simulink model "obs_student"  (R2020b)
settings: Solver=FixedStepAuto  StartTime=0.0  StopTime=Inf  FixedStep=0.01  RelTol=1e-3
model workspace (MAT data in the model file):
  SL_ROS_VariableLengthArrays_MaxSizes.CommonInfo.ArrayTruncateAction = 'EmitWarning'
  SL_ROS_VariableLengthArrays_MaxSizes.MsgTypeMap = containers.Map
  SL_ROS_VariableLengthArrays_MaxSizes.MsgTypeMap.serialization.keys = {'rcl_interfaces/ParameterValue', 'sensor_msgs/Joy', 'std_msgs/MultiArrayDimension', 'std_msgs/MultiArrayLayout'}
  SL_ROS_VariableLengthArrays_MaxSizes.MsgTypeMap.serialization.values{1}(1).PropertyName = 'bool_array_value'
  SL_ROS_VariableLengthArrays_MaxSizes.MsgTypeMap.serialization.values{1}(1).DataType = 'boolean'
  SL_ROS_VariableLengthArrays_MaxSizes.MsgTypeMap.serialization.values{1}(1).MaxLength = 128
  SL_ROS_VariableLengthArrays_MaxSizes.MsgTypeMap.serialization.values{1}(2).PropertyName = 'byte_array_value'
  SL_ROS_VariableLengthArrays_MaxSizes.MsgTypeMap.serialization.values{1}(2).DataType = 'uint8'
  SL_ROS_VariableLengthArrays_MaxSizes.MsgTypeMap.serialization.values{1}(2).MaxLength = 128
  SL_ROS_VariableLengthArrays_MaxSizes.MsgTypeMap.serialization.values{1}(3).PropertyName = 'double_array_value'
  SL_ROS_VariableLengthArrays_MaxSizes.MsgTypeMap.serialization.values{1}(3).DataType = 'double'
  SL_ROS_VariableLengthArrays_MaxSizes.MsgTypeMap.serialization.values{1}(3).MaxLength = 36
  SL_ROS_VariableLengthArrays_MaxSizes.MsgTypeMap.serialization.values{1}(4).PropertyName = 'integer_array_value'
  SL_ROS_VariableLengthArrays_MaxSizes.MsgTypeMap.serialization.values{1}(4).DataType = 'double'
  SL_ROS_VariableLengthArrays_MaxSizes.MsgTypeMap.serialization.values{1}(4).MaxLength = 128
  SL_ROS_VariableLengthArrays_MaxSizes.MsgTypeMap.serialization.values{1}(5).PropertyName = 'string_array_value'
  SL_ROS_VariableLengthArrays_MaxSizes.MsgTypeMap.serialization.values{1}(5).DataType = 'std_msgs/String'
  SL_ROS_VariableLengthArrays_MaxSizes.MsgTypeMap.serialization.values{1}(5).MaxLength = 16
  SL_ROS_VariableLengthArrays_MaxSizes.MsgTypeMap.serialization.values{1}(6).PropertyName = 'string_value'
  SL_ROS_VariableLengthArrays_MaxSizes.MsgTypeMap.serialization.values{1}(6).DataType = 'uint8'
  SL_ROS_VariableLengthArrays_MaxSizes.MsgTypeMap.serialization.values{1}(6).MaxLength = 128
  SL_ROS_VariableLengthArrays_MaxSizes.MsgTypeMap.serialization.values{2}(1).PropertyName = 'Axes'
  SL_ROS_VariableLengthArrays_MaxSizes.MsgTypeMap.serialization.values{2}(1).DataType = 'single'
  SL_ROS_VariableLengthArrays_MaxSizes.MsgTypeMap.serialization.values{2}(1).MaxLength = 20
  SL_ROS_VariableLengthArrays_MaxSizes.MsgTypeMap.serialization.values{2}(2).PropertyName = 'Buttons'
  SL_ROS_VariableLengthArrays_MaxSizes.MsgTypeMap.serialization.values{2}(2).DataType = 'int32'
  SL_ROS_VariableLengthArrays_MaxSizes.MsgTypeMap.serialization.values{2}(2).MaxLength = 17
  SL_ROS_VariableLengthArrays_MaxSizes.MsgTypeMap.serialization.values{3}.PropertyName = 'label'
  SL_ROS_VariableLengthArrays_MaxSizes.MsgTypeMap.serialization.values{3}.DataType = 'uint8'
  SL_ROS_VariableLengthArrays_MaxSizes.MsgTypeMap.serialization.values{3}.MaxLength = 2
  SL_ROS_VariableLengthArrays_MaxSizes.MsgTypeMap.serialization.values{4}.PropertyName = 'dim'
  SL_ROS_VariableLengthArrays_MaxSizes.MsgTypeMap.serialization.values{4}.DataType = 'std_msgs/MultiArrayDimension'
  SL_ROS_VariableLengthArrays_MaxSizes.MsgTypeMap.serialization.values{4}.MaxLength = 1
  SL_ROS_VariableLengthArrays_MaxSizes.MsgTypeMap.serialization.uniformity = 0
  SL_ROS_VariableLengthArrays_MaxSizes.MsgTypeMap.serialization.keyType = 'char'
  SL_ROS_VariableLengthArrays_MaxSizes.MsgTypeMap.serialization.valueType = 'any'
libraries: robotlib x6
settings Model: SILPILModeSetting=veronly  ExtModeTrigDuration=2  Creator=erlendbasso  LastModifiedBy=erlendbasso
settings OptimizationCC: EnhancedBackFolding=on  PassReuseOutputArgsAs=Individual arguments  ZeroExternalMemoryAtStartup=off  ZeroInternalMemoryAtStartup=off  MaxStackSize=64  OptimizeBlockOrder=speed  DifferentSizesBufferReuse=on  OptimizationCustomize=off  EfficientTunableParamExpr=on
settings DebuggingCC: ParameterTunabilityLossMsg=error
settings HardwareCC: ProdBitPerPointer=32  ProdBitPerSizeT=32  ProdBitPerPtrDiffT=32  ProdLargestAtomicInteger=Long  ProdLargestAtomicFloat=Double  ProdWordSize=32  ProdHWDeviceType=ARM Compatible->ARM Cortex
settings SFSimCC: SimTargetLang=C++
settings RTWCC: Description=Embedded Coder  SystemTargetFile=ert.tlc  HardwareBoard=Raspberry Pi - Robot Operating System (ROS)  TLCOptions="-aInlineSetEventsForThisBaseRateFcn=TLC_FALSE -aSuppressMultiTaskScheduler=TLC_FALSE    -aRateBasedStepFcn=0"  TemplateMakefile=ert_default_tmf  RTWUseSimCustomCode=on  Toolchain=Catkin  BuildConfiguration=Faster Runs  TargetLang=C++
settings CodeAppCC: ForceParamTrailComments=on  IgnoreCustomStorageClasses=off  OperatorAnnotations=on  SimulinkDataObjDesc=on  SFDataObjDesc=on  InsertBlockDesc=on
settings ERTTargetCC: SupportContinuousTime=on  ExtModeStaticAllocSize=250  RootIOFormat=Structure reference

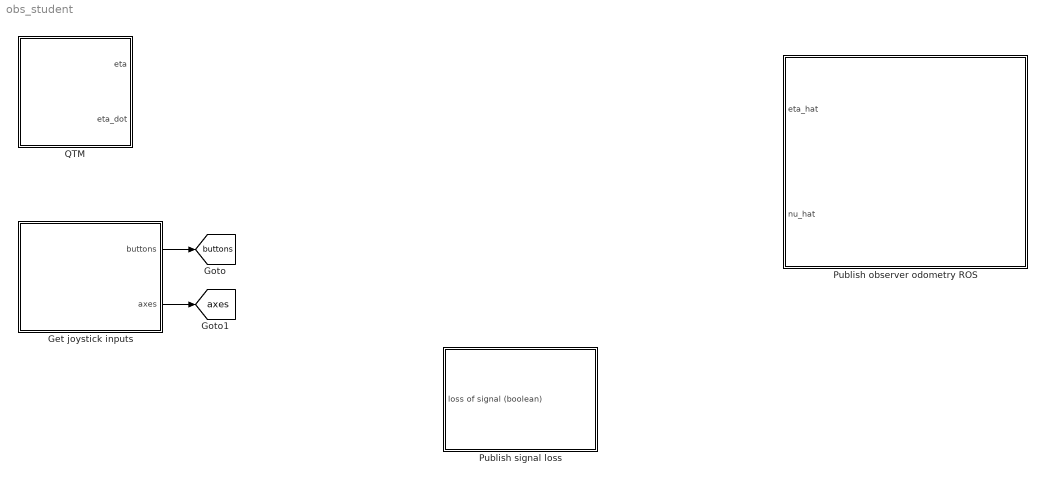
== system obs_student ==
  Get joystick inputs : Subsystem
  Publish observer odometry ROS : Subsystem
  Publish signal loss : Subsystem
  QTM : Subsystem
  tag scope: axes=global, buttons=global
  wires:
  Get joystick inputs/1(buttons) -> [buttons]
  Get joystick inputs/2(axes) -> [axes]

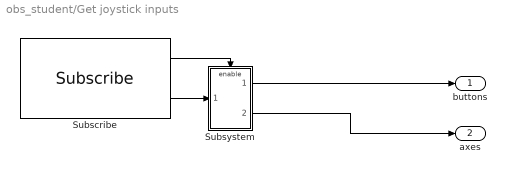
== system obs_student/Get joystick inputs ==
  Subscribe : robotlib/Subscribe  topicSource=Specify your own  topic=/joy  messageType=sensor_msgs/Joy  SampleTime=0.01  legacyBusStruct=off  messageQueueLength=1
  Subsystem : Subsystem
  buttons : Outport
  axes : Outport  Port=2
  wires:
  Subscribe/1 -> Subsystem/Enable
  Subscribe/2 -> Subsystem/1(In1)
  Subsystem/1(<Buttons>) -> buttons/1
  Subsystem/2(<Axes>) -> axes/1

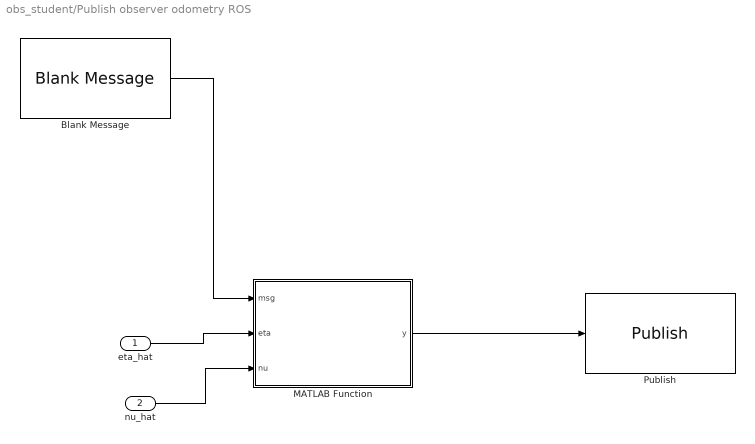
== system obs_student/Publish observer odometry ROS ==
  eta_hat : Inport
  nu_hat : Inport  Port=2
  Blank Message : robotlib/Blank Message  messageClass=Message  entityType=nav_msgs/Odometry  messageType=nav_msgs/Odometry  SampleTime=0.01  legacyBusStruct=off
  MATLAB Function : MATLAB Function  TreatAsAtomicUnit=on
  Publish : robotlib/Publish  topicSource=Specify your own  topic=/observer/odom  messageType=nav_msgs/Odometry  legacyBusStruct=off  messageQueueLength=1
  wires:
  MATLAB Function/1(y) -> Publish/1
  Blank Message/1 -> MATLAB Function/1(msg)
  eta_hat/1 -> MATLAB Function/2(eta)
  nu_hat/1 -> MATLAB Function/3(nu)

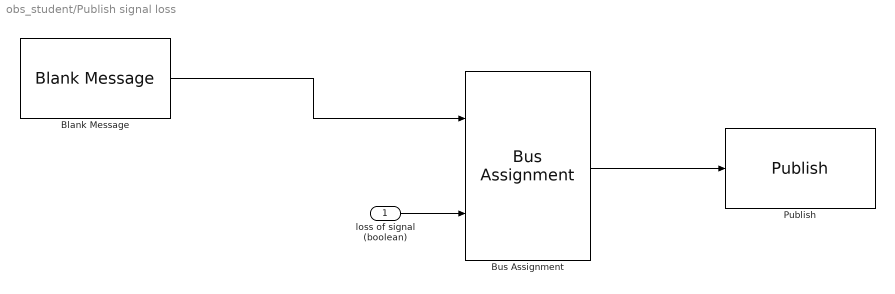
== system obs_student/Publish signal loss ==
  loss of signal (boolean) : Inport  OutDataTypeStr=boolean
  Blank Message : robotlib/Blank Message  messageClass=Message  entityType=std_msgs/Bool  messageType=std_msgs/Bool  SampleTime=0.01  legacyBusStruct=off
  Bus Assignment : BusAssignment  AssignedSignals=signal1
  Publish : robotlib/Publish  topicSource=Specify your own  topic=/CSEI/observer/errorsignal  messageType=std_msgs/Bool  legacyBusStruct=off  messageQueueLength=1
  wires:
  Blank Message/1 -> Bus Assignment/1
  Bus Assignment/1 -> Publish/1
  loss of signal (boolean)/1 -> Bus Assignment/2

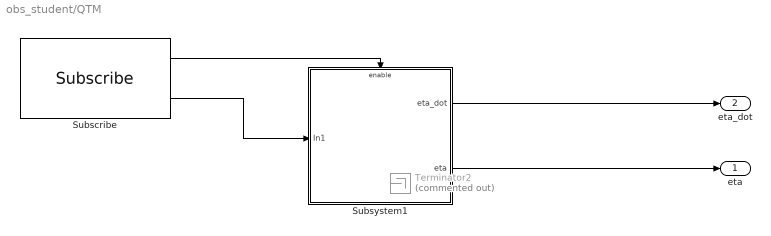
== system obs_student/QTM ==
  Subscribe : robotlib/Subscribe  topicSource=Specify your own  topic=/qualisys/CSEI/odom  messageType=nav_msgs/Odometry  SampleTime=0.01  legacyBusStruct=off  messageQueueLength=1
  Subsystem1 : Subsystem
  Terminator2 : Terminator  Commented=on
  eta : Outport
  eta_dot : Outport  Port=2
  wires:
  Subscribe/2 -> Subsystem1/1(In1)
  Subscribe/1 -> Subsystem1/Enable
  Subsystem1/1(eta_dot) -> eta_dot/1
  Subsystem1/2(eta) -> eta/1

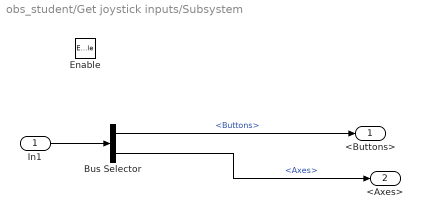
== system obs_student/Get joystick inputs/Subsystem ==
  In1 : Inport
  Enable : EnablePort
  Bus Selector : BusSelector  OutputSignals=Buttons,Axes
  <Buttons> : Outport
  <Axes> : Outport  Port=2
  wires:
  In1/1 -> Bus Selector/1
  Bus Selector/1 -> <Buttons>/1  "<Buttons>"
  Bus Selector/2 -> <Axes>/1  "<Axes>"

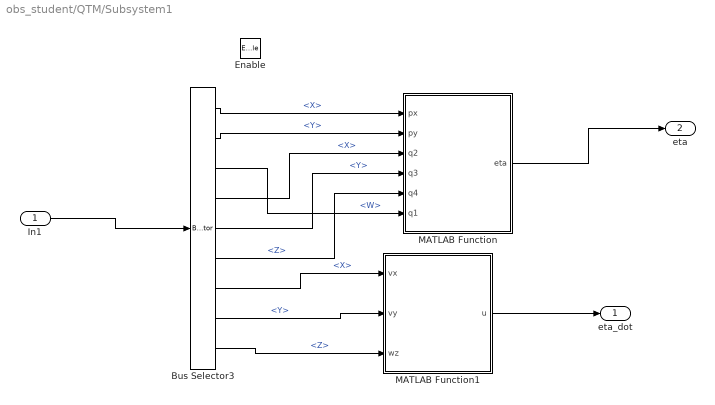
== system obs_student/QTM/Subsystem1 ==
  In1 : Inport
  Enable : EnablePort
  Bus Selector3 : BusSelector  OutputSignals=Pose.Pose.Position.X,Pose.Pose.Position.Y,Pose.Pose.Orientation.W,Pose.Pose.Orientation.X,Pose.Pose.Orientation.Y,Pose.Pose.Orientation.Z,Twist.Twist.Linear.X,Twist.Twist.Linear.Y,Twist.Twist.Angular.Z
  MATLAB Function : MATLAB Function  TreatAsAtomicUnit=on
  MATLAB Function1 : MATLAB Function  TreatAsAtomicUnit=on
  eta_dot : Outport
  eta : Outport  Port=2
  wires:
  In1/1 -> Bus Selector3/1
  MATLAB Function1/1(u) -> eta_dot/1
  Bus Selector3/7 -> MATLAB Function1/1(vx)  "<X>"
  Bus Selector3/8 -> MATLAB Function1/2(vy)  "<Y>"
  Bus Selector3/9 -> MATLAB Function1/3(wz)  "<Z>"
  MATLAB Function/1(eta) -> eta/1
  Bus Selector3/1 -> MATLAB Function/1(px)  "<X>"
  Bus Selector3/2 -> MATLAB Function/2(py)  "<Y>"
  Bus Selector3/3 -> MATLAB Function/6(q1)  "<W>"
  Bus Selector3/4 -> MATLAB Function/3(q2)  "<X>"
  Bus Selector3/5 -> MATLAB Function/4(q3)  "<Y>"
  Bus Selector3/6 -> MATLAB Function/5(q4)  "<Z>"

== matlab function obs_student/Publish observer odometry ROS/MATLAB Function ==
  data: msg input; eta input; y output Bus: SL_Bus_CSEI_HIL_ros_nav_msgs_Odometry; nu input
function y = fcn(msg,eta,nu)

y = msg;

quat = eul2quat([0 0 eta(3)], 'XYZ');

y.Pose.Pose.Position.X = eta(1);
y.Pose.Pose.Position.Y = eta(2);
y.Pose.Pose.Position.Z = 0;
y.Pose.Pose.Orientation.W = quat(1);
y.Pose.Pose.Orientation.X = quat(2);
y.Pose.Pose.Orientation.Y = quat(3);
y.Pose.Pose.Orientation.Z = quat(4);


y.Twist.Twist.Linear.X = nu(1);
y.Twist.Twist.Linear.Y = nu(2);
y.Twist.Twist.Linear.Z = 0;
y.Twist.Twist.Angular.X = 0;
y.Twist.Twist.Angular.Y = 0;
y.Twist.Twist.Angular.Z = nu(3);

== matlab function obs_student/QTM/Subsystem1/MATLAB Function1 ==
  data: vx input; u output; vy input; wz input
function u = fcn(vx,vy,wz)

u = [vx;vy;wz];

== matlab function obs_student/QTM/Subsystem1/MATLAB Function ==
  data: px input; eta output; py input; q2 input; q3 input; q4 input; q1 input
function eta = fcn(px,py,q2,q3,q4,q1)

quat = [q1;q2;q3;q4];
eul = quat2eul(quat','XYZ');

eta = [px;py;eul(3)];
